simulink model "RedAsociativa"  (Simulink 8.7)
settings: Solver=ode45  StartTime=0.0  StopTime=10.0  RelTol=1e-3
settings Model: Creator=My Laptop  LastModifiedBy=Mariano
settings DataIOCC: SignalLoggingSaveFormat=ModelDataLogs
settings OptimizationCC: ExpressionDepthLimit=2147483647
settings DebuggingCC: SolverPrmCheckMsg=warning  FcnCallInpInsideContextMsg=UseLocalSettings  StateNameClashWarn=warning
settings GRTTargetCC: CombineOutputUpdateFcns=off  GRTInterface=on

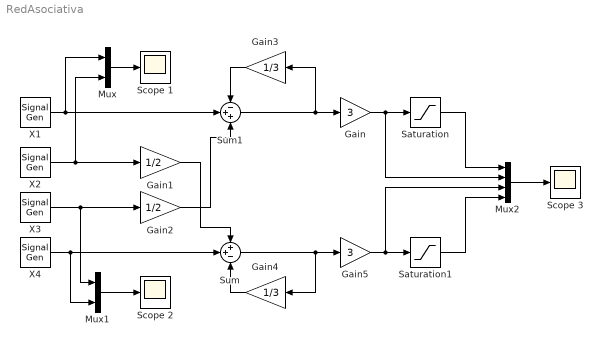
== system RedAsociativa ==
  Gain : Gain  Gain=3
  Gain1 : Gain  Gain=1/2
  Gain2 : Gain  Gain=1/2
  Gain3 : Gain  Gain=1/3
  Gain4 : Gain  Gain=1/3
  Gain5 : Gain  Gain=3
  Mux : Mux  Inputs=2
  Mux1 : Mux  Inputs=2
  Mux2 : Mux
  Saturation : Saturate  UpperLimit=1  LowerLimit=-1  ZeroCross=off
  Saturation1 : Saturate  UpperLimit=1  LowerLimit=-1  ZeroCross=off
  Scope 1 : Scope
  Scope 2 : Scope
  Scope 3 : Scope
  Sum : Sum  Inputs=++-
  Sum1 : Sum  Inputs=-++
  X1 : SignalGenerator  WaveForm=square  Frequency=.8
  X2 : SignalGenerator  WaveForm=square  Frequency=.4
  X3 : SignalGenerator  WaveForm=square  Frequency=.2
  X4 : SignalGenerator  WaveForm=square  Frequency=.1
  wires:
  Mux/1 -> Scope 1/1
  X1/1 -> Mux/1, Sum1/2
  X2/1 -> Mux/2, Gain1/1
  Mux1/1 -> Scope 2/1
  X3/1 -> Mux1/1, Gain2/1
  X4/1 -> Mux1/2, Sum/2
  Gain3/1 -> Sum1/1
  Sum1/1 -> Gain3/1, Gain/1
  Gain4/1 -> Sum/3
  Sum/1 -> Gain4/1, Gain5/1
  Gain2/1 -> Sum1/3
  Gain1/1 -> Sum/1
  Mux2/1 -> Scope 3/1
  Gain/1 -> Saturation/1, Mux2/2
  Gain5/1 -> Saturation1/1, Mux2/3
  Saturation/1 -> Mux2/1
  Saturation1/1 -> Mux2/4
